simulink subsystem "L289N_IN1_IN2"  (R2024a)
settings: Solver=VariableStepAuto  StartTime=0.0  StopTime=10.0  RelTol=1e-3
settings Model: Creator=Peter  LastModifiedBy=Peter

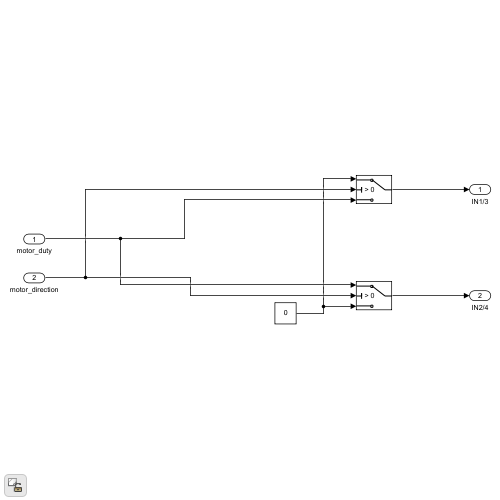
[thumbnail: Simulink's stored preview of the top-level diagram]
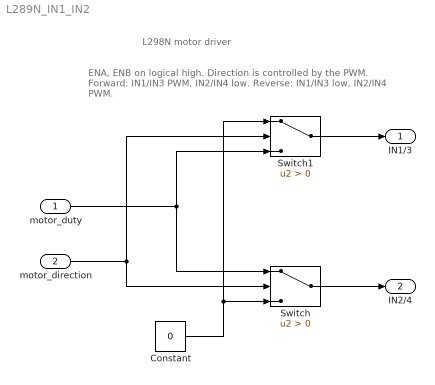
== system L289N_IN1_IN2 ==
  note: ENA, ENB on logical high. Direction is controlled by the PWM.
      | Forward: IN1/IN3 PWM, IN2/IN4 low.
      | Reverse: IN1/IN3 low, IN2/IN4 PWM.
  note: L298N motor driver
  motor_duty : Inport
  motor_direction : Inport  Port=2
  Constant : Constant  Value=0  OutDataTypeStr=single
  Switch : Switch  Criteria=u2 > Threshold  SaturateOnIntegerOverflow=off  InputSameDT=off
  Switch1 : Switch  Criteria=u2 > Threshold  SaturateOnIntegerOverflow=off  InputSameDT=off
  IN1/3 : Outport
  IN2/4 : Outport  Port=2
  wires:
  Constant/1 -> Switch/3, Switch1/1
  motor_direction/1 -> Switch1/2, Switch/2
  motor_duty/1 -> Switch1/3, Switch/1
  Switch1/1 -> IN1/3/1
  Switch/1 -> IN2/4/1
